simulink model "TP_ex3"  (R2020b)
settings: Solver=VariableStepAuto  StartTime=0.0  StopTime=10.0  RelTol=1e-3
settings Model: Creator=macbook  LastModifiedBy=macbook

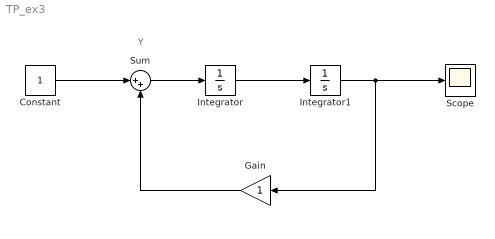
== system TP_ex3 ==
  note: Y
  Constant : Constant
  Gain : Gain
  Integrator : Integrator
  Integrator1 : Integrator
  Scope : Scope
  Sum : Sum  Inputs=|++
  wires:
  Constant/1 -> Sum/1
  Integrator1/1 -> Gain/1, Scope/1
  Integrator/1 -> Integrator1/1
  Sum/1 -> Integrator/1
  Gain/1 -> Sum/2
